simulink model "PFC_69C_03_06_V01_3Phase_3_2KW"  (R2022b)
settings: Solver=FixedStepAuto  StartTime=0.0  StopTime=Inf  RelTol=1e-3  EnableMultiTasking=on
model workspace (MAT data in the model file):
  ADC_Gain = 1241.21212121
  DAC_Gain = 0.000805860805861
  Inductor_Current_Divider_Gain_Phase_A = 33.4
  Inductor_Current_Divider_Gain_Phase_B = 33.4
  Vbulk_Divider_Gain = 276.854928018
  Vin_Divider_Gain = 556.17352614
undefined symbols (not defined in the file or in its folder): GPTRIP1SEL, GPTRIP2SEL, SCI_A_Transmit, SCI_A_Transmit_Current_Suffix, SCI_A_Transmit_one_shot_Suffix, SCI_A_Transmit_Polarity_Suffix, SCI_A_Transmit_relay_Suffix, SCI_A_Transmit_Vbulk_Suffix, SCI_A_Transmit_Vin_rms_Suffix, SCI_A_Transmit_Vin_Suffix, SCI_A_Transmit_Vmid_Suffix, SCI_A_Transmit_Vp_Suffix, SCI_A_Transmit_Vpfc_Suffix, TZ1, TZ2
libraries: c280xlib x38, c2802xlib x34, simulink x17, c2000lib x1
(part 2 of 8)

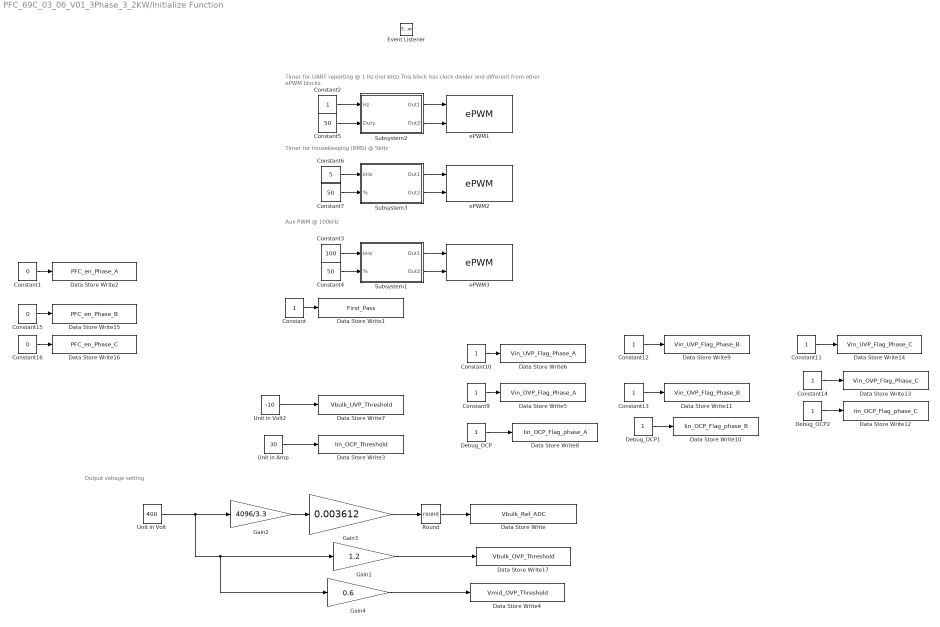
== system PFC_69C_03_06_V01_3Phase_3_2KW/Initialize Function ==
  note: Aux PWM @ 100kHz
  note: Timer for UART reporting @ 1 Hz (not kHz)
      | This block has clock divider and different from other ePWM blocks.
  note: Timer for housekeeping (RMS) @ 5kHz
  note: Output voltage setting
  Constant{,2,9..14} (8 alike) : Constant
  Constant1 : Constant  Value=0
  Constant15 : Constant  Value=0
  Constant16 : Constant  Value=0
  Constant3 : Constant  Value=100
  Constant4 : Constant  Value=50
  Constant5 : Constant  Value=50
  Constant6 : Constant  Value=5
  Constant7 : Constant  Value=50
  Data Store Write : DataStoreWrite  DataStoreName=Vbulk_Ref_ADC  IndexOptions=Index vector (dialog)  Indices=1  OutputSizes=1
  Data Store Write1 : DataStoreWrite  DataStoreName=First_Pass  IndexOptions=Index vector (dialog)  Indices=1  OutputSizes=1
  Data Store Write10 : DataStoreWrite  DataStoreName=Iin_OCP_Flag_phase_B  IndexOptions=Index vector (dialog)  Indices=1  OutputSizes=1
  Data Store Write11 : DataStoreWrite  DataStoreName=Vin_OVP_Flag_Phase_B  IndexOptions=Index vector (dialog)  Indices=1  OutputSizes=1
  Data Store Write12 : DataStoreWrite  DataStoreName=Iin_OCP_Flag_phase_C  IndexOptions=Index vector (dialog)  Indices=1  OutputSizes=1
  Data Store Write13 : DataStoreWrite  DataStoreName=Vin_OVP_Flag_Phase_C  IndexOptions=Index vector (dialog)  Indices=1  OutputSizes=1
  Data Store Write14 : DataStoreWrite  DataStoreName=Vin_UVP_Flag_Phase_C  IndexOptions=Index vector (dialog)  Indices=1  OutputSizes=1
  Data Store Write15 : DataStoreWrite  DataStoreName=PFC_en_Phase_B  IndexOptions=Index vector (dialog)  Indices=1  OutputSizes=1
  Data Store Write16 : DataStoreWrite  DataStoreName=PFC_en_Phase_C  IndexOptions=Index vector (dialog)  Indices=1  OutputSizes=1
  Data Store Write17 : DataStoreWrite  DataStoreName=Vbulk_OVP_Threshold  IndexOptions=Index vector (dialog)  Indices=1  OutputSizes=1
  Data Store Write2 : DataStoreWrite  DataStoreName=PFC_en_Phase_A  IndexOptions=Index vector (dialog)  Indices=1  OutputSizes=1
  Data Store Write3 : DataStoreWrite  DataStoreName=Iin_OCP_Threshold  IndexOptions=Index vector (dialog)  Indices=1  OutputSizes=1
  Data Store Write4 : DataStoreWrite  DataStoreName=Vmid_OVP_Threshold  IndexOptions=Index vector (dialog)  Indices=1  OutputSizes=1
  Data Store Write5 : DataStoreWrite  DataStoreName=Vin_OVP_Flag_Phase_A  IndexOptions=Index vector (dialog)  Indices=1  OutputSizes=1
  Data Store Write6 : DataStoreWrite  DataStoreName=Vin_UVP_Flag_Phase_A  IndexOptions=Index vector (dialog)  Indices=1  OutputSizes=1
  Data Store Write7 : DataStoreWrite  DataStoreName=Vbulk_UVP_Threshold  IndexOptions=Index vector (dialog)  Indices=1  OutputSizes=1
  Data Store Write8 : DataStoreWrite  DataStoreName=Iin_OCP_Flag_phase_A  IndexOptions=Index vector (dialog)  Indices=1  OutputSizes=1
  Data Store Write9 : DataStoreWrite  DataStoreName=Vin_UVP_Flag_Phase_B  IndexOptions=Index vector (dialog)  Indices=1  OutputSizes=1
  Debug_OCP : Constant
  Debug_OCP1 : Constant
  Debug_OCP2 : Constant
  Event Listener : EventListener  DisableCoverage=on  EventName=reset
  Gain1 : Gain  Gain=1.2
  Gain2 : Gain  Gain=4096/3.3
  Gain3 : Gain  Gain=0.003612  OutDataTypeStr=double
  Gain4 : Gain  Gain=0.6
  Round : Rounding  Operator=round
  Subsystem1 : Subsystem
  Subsystem2 : Subsystem
  Subsystem3 : Subsystem
  Unit in Amp : Constant  Value=30
  Unit in Volt : Constant  Value=400
  Unit in Volt2 : Constant  Value=-10
  ePWM1 : c2802xlib/ePWM  PwmType=C2000  useModule=ePWM7  ePWMxLINKTBPRD=Not Linked  periodUnits=Clock cycles  timerSource=Input port  timerPeriod_clk=50224  timerPeriod_sec=0.0001  tbshadow=Counter equals to zero  countingMode=Up  phaseActiveEnable=Disable  phaseDirection=Count down after sync  phaseActive=0  synchronizationEnable=off  dcaevt1Sync=off  dcbevt1Sync=off  synchronizationOption=Disable  dcbevt1SyncOut=off  dcaevt1SyncOut=off  cmpdSyncOut=off  cmpcSyncOut=off  cmpbSyncOut=off  zeroSyncOut=off  swfSyncOut=off  perSynchronizationOption=Counter equals to period (CTR=PRD)  clockPrescale=128  HSclockPrescale=14  enswap=off  ePWMxAStatus=on  ePWMxAactionLogic1=Clear  ePWMxAactionLogic2=Do nothing  ePWMxAactionLogic3=Set  ePWMxAactionLogic4=Set  ePWMxAactionLogic5=Do nothing  ePWMxAactionLogic6=Do nothing  ePWMxACSFenable=off  ePWMxACSFvalue=Forcing disable  ePWMxASFreload=Zero  ePWMxBStatus=off  ePWMxBactionLogic1=Set  ePWMxBactionLogic2=Do nothing  ePWMxBactionLogic3=Clear  ePWMxBactionLogic4=Do nothing  ePWMxBactionLogic5=Do nothing  ePWMxBactionLogic6=Set  ePWMxBCSFenable=off  ePWMxBCSFvalue=Forcing disable  ePWMxBSFreload=Zero  ePWNxBOutWay=off  ePWMxLINKCMPA=Not Linked  CMPAUnits=Clock cycles  CMPASource=Input port  CMPAValue_per=50  CMPAValue_clk=32000  enCMPAshadow=Counter equals to zero (CTR=Zero)  ePWMxLINKCMPB=Not Linked  CMPBUnits=Clock cycles  CMPBSource=Specify via dialog  CMPBValue_per=50  CMPBValue_clk=32000  enCMPBshadow=Counter equals to zero (CTR=Zero)  ePWMxLINKCMPC=Not Linked  CMPCUnits=Clock cycles  CMPCSource=Specify via dialog  CMPCValue_per=50  CMPCValue_clk=32000  enCMPCshadow=Counter equals to zero (CTR=Zero)  ePWMxLINKCMPD=Not Linked  CMPDUnits=Clock cycles  CMPDSource=Specify via dialog  CMPDValue_per=50  CMPDValue_clk=32000  enCMPDshadow=Counter equals to zero (CTR=Zero)  enableDBePWMxA=off  enableDBePWMxB=off  enhalfcycle=off  DBpolarity=Active high (AH)  DBedgeDelay=Positive  DBSource_ePWMxA=ePWMxA  DBSource_ePWMxB=ePWMxA  DBPeriodUnits=Clock cycles  DBperiodSource=Specify via dialog  REDperiod=0  FEDperiod=0  REDperiod_sec=0  FEDperiod_sec=0  LoadModeDBRED=Immediate without using shadow  LoadModeDBFED=Immediate without using shadow  adcstartModuleA=off  adcrequestEventA=First event  adcstartEventA=Counter equals to zero (CTR=Zero)  adcstartEventA_type2=Digital Compare Module A Event 1 start of conversion (DCAEVT1.soc)  adcstartModuleB=off  adcrequestEventB=First event  adcstartEventB=Counter equals to zero (CTR=Zero)  adcstartEventB_type2=Counter equals to zero (CTR=Zero)  intEn=on  intPrd=First event  intSel=Counter equals to zero (CTR=Zero)  intSel_type2=Counter equals to zero (CTR=Zero)  hrpe=off  enHRPWM=off  HRPWM_LoadMode=Counter equals to period (CTR=PRD)  HRPWM_CTLMode=Duty or Period control mode  HRPWM_EDGMode=Both edge  hrpeb=off  enHRPWMB=off  HRPWM_LoadModeB=Counter equals to zero (CTR=ZERO)  HRPWM_CTLModeB=Duty or Period control mode  HRPWM_EDGModeB=Both edge  enHRDBRED=off  enHRDBFED=off  enSFO=on  enautoconv=on  chopperEnable=off  chopperFrequency=1  chopperFirstwidth=1  chopperDuty=12.5%  tripZonesource=Specify via dialog  tzselOSHT1=off  tzselOSHT2=off  tzselOSHT3=off  tzselOSHDCAEV1=off  tzselOSHDCBEV1=off  tzselCBC1=off  tzselCBC2=off  tzselCBC3=off  tzselCBCDCAEV2=off  tzselCBCDCBEV2=off  tzselOSHT4=off  tzselOSHT5=off  tzselOSHT6=off  tzselCBC4=off  tzselCBC5=off  tzselCBC6=off  enTzOstIntr=off  enTzCbcIntr=off  enTzDCAEVT1Intr=off  enTzDCAEVT2Intr=off  enTzDCBEVT1Intr=off  enTzDCBEVT2Intr=off  ePWMxAforced=No action  ePWMxBforced=No action  DCAEVT1forced=No action  DCBEVT1forced=No action  DCAEVT2forced=No action  DCBEVT2forced=No action  dcah=Trip Zone 1 input (TZ1)  dcal=Trip Zone 1 input (TZ1)  dcbh=Trip Zone 1 input (TZ1)  dcbl=Trip Zone 1 input (TZ1)  dcah_type2=GPTRIP1SEL/(TZ1)  dcal_type2=GPTRIP2SEL/(TZ2)  dcbh_type2=GPTRIP1SEL/(TZ1)  dcbl_type2=GPTRIP2SEL/(TZ2)  gendcaevt1=Event disabled  gendcaevt2=Event disabled  gendcbevt1=Event disabled  gendcbevt2=Event disabled  dcaevt1src=DCAEVT1 with sync  dcaevt2src=DCAEVT2 with sync  dcbevt1src=DCBEVT1 with sync  dcbevt2src=DCBEVT2 with sync  pulsesel=Counter equals to zero (CTR=Zero)  blankinv=off  blankoffset=0  blankwidth=0  evsrcsel=Filtered version of DCAEVT1 (DCAEVT1FILT)  encape=off
      settings: LibrarySourceBlock=c2806xlib/ePWM
  ePWM2 : c2802xlib/ePWM  PwmType=C2000  useModule=ePWM4  ePWMxLINKTBPRD=Not Linked  periodUnits=Clock cycles  timerSource=Input port  timerPeriod_clk=64000  timerPeriod_sec=0.0001  tbshadow=Counter equals to zero  countingMode=Up  phaseActiveEnable=Disable  phaseDirection=Count down after sync  phaseActive=0  synchronizationEnable=off  dcaevt1Sync=off  dcbevt1Sync=off  synchronizationOption=Disable  dcbevt1SyncOut=off  dcaevt1SyncOut=off  cmpdSyncOut=off  cmpcSyncOut=off  cmpbSyncOut=off  zeroSyncOut=off  swfSyncOut=off  perSynchronizationOption=Counter equals to period (CTR=PRD)  clockPrescale=1  HSclockPrescale=1  enswap=off  ePWMxAStatus=on  ePWMxAactionLogic1=Clear  ePWMxAactionLogic2=Do nothing  ePWMxAactionLogic3=Set  ePWMxAactionLogic4=Set  ePWMxAactionLogic5=Do nothing  ePWMxAactionLogic6=Do nothing  ePWMxACSFenable=off  ePWMxACSFvalue=Forcing disable  ePWMxASFreload=Zero  ePWMxBStatus=off  ePWMxBactionLogic1=Set  ePWMxBactionLogic2=Do nothing  ePWMxBactionLogic3=Clear  ePWMxBactionLogic4=Do nothing  ePWMxBactionLogic5=Do nothing  ePWMxBactionLogic6=Set  ePWMxBCSFenable=off  ePWMxBCSFvalue=Forcing disable  ePWMxBSFreload=Zero  ePWNxBOutWay=off  ePWMxLINKCMPA=Not Linked  CMPAUnits=Clock cycles  CMPASource=Input port  CMPAValue_per=50  CMPAValue_clk=32000  enCMPAshadow=Counter equals to zero (CTR=Zero)  ePWMxLINKCMPB=Not Linked  CMPBUnits=Clock cycles  CMPBSource=Specify via dialog  CMPBValue_per=50  CMPBValue_clk=32000  enCMPBshadow=Counter equals to zero (CTR=Zero)  ePWMxLINKCMPC=Not Linked  CMPCUnits=Clock cycles  CMPCSource=Specify via dialog  CMPCValue_per=50  CMPCValue_clk=32000  enCMPCshadow=Counter equals to zero (CTR=Zero)  ePWMxLINKCMPD=Not Linked  CMPDUnits=Clock cycles  CMPDSource=Specify via dialog  CMPDValue_per=50  CMPDValue_clk=32000  enCMPDshadow=Counter equals to zero (CTR=Zero)  enableDBePWMxA=off  enableDBePWMxB=off  enhalfcycle=off  DBpolarity=Active high (AH)  DBedgeDelay=Positive  DBSource_ePWMxA=ePWMxA  DBSource_ePWMxB=ePWMxA  DBPeriodUnits=Clock cycles  DBperiodSource=Specify via dialog  REDperiod=0  FEDperiod=0  REDperiod_sec=0  FEDperiod_sec=0  LoadModeDBRED=Immediate without using shadow  LoadModeDBFED=Immediate without using shadow  adcstartModuleA=off  adcrequestEventA=First event  adcstartEventA=Counter equals to zero (CTR=Zero)  adcstartEventA_type2=Digital Compare Module A Event 1 start of conversion (DCAEVT1.soc)  adcstartModuleB=off  adcrequestEventB=First event  adcstartEventB=Counter equals to zero (CTR=Zero)  adcstartEventB_type2=Counter equals to zero (CTR=Zero)  intEn=on  intPrd=First event  intSel=Counter equals to zero (CTR=Zero)  intSel_type2=Counter equals to zero (CTR=Zero)  hrpe=off  enHRPWM=off  HRPWM_LoadMode=Counter equals to period (CTR=PRD)  HRPWM_CTLMode=Duty or Period control mode  HRPWM_EDGMode=Both edge  hrpeb=off  enHRPWMB=off  HRPWM_LoadModeB=Counter equals to zero (CTR=ZERO)  HRPWM_CTLModeB=Duty or Period control mode  HRPWM_EDGModeB=Both edge  enHRDBRED=off  enHRDBFED=off  enSFO=on  enautoconv=on  chopperEnable=off  chopperFrequency=1  chopperFirstwidth=1  chopperDuty=12.5%  tripZonesource=Specify via dialog  tzselOSHT1=off  tzselOSHT2=off  tzselOSHT3=off  tzselOSHDCAEV1=off  tzselOSHDCBEV1=off  tzselCBC1=off  tzselCBC2=off  tzselCBC3=off  tzselCBCDCAEV2=off  tzselCBCDCBEV2=off  tzselOSHT4=off  tzselOSHT5=off  tzselOSHT6=off  tzselCBC4=off  tzselCBC5=off  tzselCBC6=off  enTzOstIntr=off  enTzCbcIntr=off  enTzDCAEVT1Intr=off  enTzDCAEVT2Intr=off  enTzDCBEVT1Intr=off  enTzDCBEVT2Intr=off  ePWMxAforced=No action  ePWMxBforced=No action  DCAEVT1forced=No action  DCBEVT1forced=No action  DCAEVT2forced=No action  DCBEVT2forced=No action  dcah=Trip Zone 1 input (TZ1)  dcal=Trip Zone 1 input (TZ1)  dcbh=Trip Zone 1 input (TZ1)  dcbl=Trip Zone 1 input (TZ1)  dcah_type2=GPTRIP1SEL/(TZ1)  dcal_type2=GPTRIP2SEL/(TZ2)  dcbh_type2=GPTRIP1SEL/(TZ1)  dcbl_type2=GPTRIP2SEL/(TZ2)  gendcaevt1=Event disabled  gendcaevt2=Event disabled  gendcbevt1=Event disabled  gendcbevt2=Event disabled  dcaevt1src=DCAEVT1 with sync  dcaevt2src=DCAEVT2 with sync  dcbevt1src=DCBEVT1 with sync  dcbevt2src=DCBEVT2 with sync  pulsesel=Counter equals to zero (CTR=Zero)  blankinv=off  blankoffset=0  blankwidth=0  evsrcsel=Filtered version of DCAEVT1 (DCAEVT1FILT)  encape=off
      settings: LibrarySourceBlock=c2806xlib/ePWM
  ePWM3 : c2802xlib/ePWM  PwmType=C2000  useModule=ePWM8  ePWMxLINKTBPRD=Not Linked  periodUnits=Clock cycles  timerSource=Input port  timerPeriod_clk=64000  timerPeriod_sec=0.0001  tbshadow=Counter equals to zero  countingMode=Up  phaseActiveEnable=Disable  phaseDirection=Count down after sync  phaseActive=0  synchronizationEnable=off  dcaevt1Sync=off  dcbevt1Sync=off  synchronizationOption=Disable  dcbevt1SyncOut=off  dcaevt1SyncOut=off  cmpdSyncOut=off  cmpcSyncOut=off  cmpbSyncOut=off  zeroSyncOut=off  swfSyncOut=off  perSynchronizationOption=Counter equals to period (CTR=PRD)  clockPrescale=1  HSclockPrescale=1  enswap=off  ePWMxAStatus=on  ePWMxAactionLogic1=Clear  ePWMxAactionLogic2=Do nothing  ePWMxAactionLogic3=Set  ePWMxAactionLogic4=Set  ePWMxAactionLogic5=Do nothing  ePWMxAactionLogic6=Do nothing  ePWMxACSFenable=off  ePWMxACSFvalue=Forcing disable  ePWMxASFreload=Zero  ePWMxBStatus=on  ePWMxBactionLogic1=Set  ePWMxBactionLogic2=Do nothing  ePWMxBactionLogic3=Clear  ePWMxBactionLogic4=Do nothing  ePWMxBactionLogic5=Do nothing  ePWMxBactionLogic6=Set  ePWMxBCSFenable=off  ePWMxBCSFvalue=Forcing disable  ePWMxBSFreload=Zero  ePWNxBOutWay=off  ePWMxLINKCMPA=Not Linked  CMPAUnits=Clock cycles  CMPASource=Input port  CMPAValue_per=50  CMPAValue_clk=32000  enCMPAshadow=Counter equals to zero (CTR=Zero)  ePWMxLINKCMPB=Not Linked  CMPBUnits=Clock cycles  CMPBSource=Specify via dialog  CMPBValue_per=50  CMPBValue_clk=32000  enCMPBshadow=Counter equals to zero (CTR=Zero)  ePWMxLINKCMPC=Not Linked  CMPCUnits=Clock cycles  CMPCSource=Specify via dialog  CMPCValue_per=50  CMPCValue_clk=32000  enCMPCshadow=Counter equals to zero (CTR=Zero)  ePWMxLINKCMPD=Not Linked  CMPDUnits=Clock cycles  CMPDSource=Specify via dialog  CMPDValue_per=50  CMPDValue_clk=32000  enCMPDshadow=Counter equals to zero (CTR=Zero)  enableDBePWMxA=off  enableDBePWMxB=off  enhalfcycle=off  DBpolarity=Active high (AH)  DBedgeDelay=Positive  DBSource_ePWMxA=ePWMxA  DBSource_ePWMxB=ePWMxA  DBPeriodUnits=Clock cycles  DBperiodSource=Specify via dialog  REDperiod=0  FEDperiod=0  REDperiod_sec=0  FEDperiod_sec=0  LoadModeDBRED=Immediate without using shadow  LoadModeDBFED=Immediate without using shadow  adcstartModuleA=off  adcrequestEventA=First event  adcstartEventA=Counter equals to zero (CTR=Zero)  adcstartEventA_type2=Digital Compare Module A Event 1 start of conversion (DCAEVT1.soc)  adcstartModuleB=off  adcrequestEventB=First event  adcstartEventB=Counter equals to zero (CTR=Zero)  adcstartEventB_type2=Counter equals to zero (CTR=Zero)  intEn=off  intPrd=First event  intSel=Counter equals to zero (CTR=Zero)  intSel_type2=Counter equals to zero (CTR=Zero)  hrpe=off  enHRPWM=off  HRPWM_LoadMode=Counter equals to period (CTR=PRD)  HRPWM_CTLMode=Duty or Period control mode  HRPWM_EDGMode=Both edge  hrpeb=off  enHRPWMB=off  HRPWM_LoadModeB=Counter equals to zero (CTR=ZERO)  HRPWM_CTLModeB=Duty or Period control mode  HRPWM_EDGModeB=Both edge  enHRDBRED=off  enHRDBFED=off  enSFO=on  enautoconv=on  chopperEnable=off  chopperFrequency=1  chopperFirstwidth=1  chopperDuty=12.5%  tripZonesource=Specify via dialog  tzselOSHT1=off  tzselOSHT2=off  tzselOSHT3=off  tzselOSHDCAEV1=off  tzselOSHDCBEV1=off  tzselCBC1=off  tzselCBC2=off  tzselCBC3=off  tzselCBCDCAEV2=off  tzselCBCDCBEV2=off  tzselOSHT4=off  tzselOSHT5=off  tzselOSHT6=off  tzselCBC4=off  tzselCBC5=off  tzselCBC6=off  enTzOstIntr=off  enTzCbcIntr=off  enTzDCAEVT1Intr=off  enTzDCAEVT2Intr=off  enTzDCBEVT1Intr=off  enTzDCBEVT2Intr=off  ePWMxAforced=No action  ePWMxBforced=No action  DCAEVT1forced=No action  DCBEVT1forced=No action  DCAEVT2forced=No action  DCBEVT2forced=No action  dcah=Trip Zone 1 input (TZ1)  dcal=Trip Zone 1 input (TZ1)  dcbh=Trip Zone 1 input (TZ1)  dcbl=Trip Zone 1 input (TZ1)  dcah_type2=GPTRIP1SEL/(TZ1)  dcal_type2=GPTRIP2SEL/(TZ2)  dcbh_type2=GPTRIP1SEL/(TZ1)  dcbl_type2=GPTRIP2SEL/(TZ2)  gendcaevt1=Event disabled  gendcaevt2=Event disabled  gendcbevt1=Event disabled  gendcbevt2=Event disabled  dcaevt1src=DCAEVT1 with sync  dcaevt2src=DCAEVT2 with sync  dcbevt1src=DCBEVT1 with sync  dcbevt2src=DCBEVT2 with sync  pulsesel=Counter equals to zero (CTR=Zero)  blankinv=off  blankoffset=0  blankwidth=0  evsrcsel=Filtered version of DCAEVT1 (DCAEVT1FILT)  encape=off
      settings: LibrarySourceBlock=c2806xlib/ePWM
  wires:
  Constant6/1 -> Subsystem3/1(kHz)
  Constant7/1 -> Subsystem3/2(%)
  Constant4/1 -> Subsystem1/2(%)
  Subsystem1/1(Out1) -> ePWM3/1
  Constant2/1 -> Subsystem2/1(Hz)
  Subsystem3/2(Out2) -> ePWM2/2
  Subsystem3/1(Out1) -> ePWM2/1
  Constant3/1 -> Subsystem1/1(kHz)
  Constant5/1 -> Subsystem2/2(Duty)
  Subsystem2/1(Out1) -> ePWM1/1
  Subsystem1/2(Out2) -> ePWM3/2
  Subsystem2/2(Out2) -> ePWM1/2
  Constant/1 -> Data Store Write1/1
  Constant1/1 -> Data Store Write2/1
  Gain2/1 -> Gain3/1
  Constant9/1 -> Data Store Write5/1
  Constant10/1 -> Data Store Write6/1
  Unit in Volt2/1 -> Data Store Write7/1
  Unit in Amp/1 -> Data Store Write3/1
  Debug_OCP/1 -> Data Store Write8/1
  Gain3/1 -> Round/1
  Round/1 -> Data Store Write/1
  Constant12/1 -> Data Store Write9/1
  Debug_OCP1/1 -> Data Store Write10/1
  Constant13/1 -> Data Store Write11/1
  Debug_OCP2/1 -> Data Store Write12/1
  Constant14/1 -> Data Store Write13/1
  Constant11/1 -> Data Store Write14/1
  Constant15/1 -> Data Store Write15/1
  Constant16/1 -> Data Store Write16/1
  Gain1/1 -> Data Store Write17/1
  Unit in Volt/1 -> Gain4/1, Gain1/1, Gain2/1
  Gain4/1 -> Data Store Write4/1

== system PFC_69C_03_06_V01_3Phase_3_2KW/Initialize ePWM1 ==

== system PFC_69C_03_06_V01_3Phase_3_2KW/PWM Update @50KHz ==
  note: This block will update PWM after control calculations.==>
  function : TriggerPort  TriggerType=function-call  VariantControl=(inherit)
  Current loop PWM generation (Control) : Subsystem  TreatAsAtomicUnit=on
  Fixed Duty update_Phase_A : Subsystem  TreatAsAtomicUnit=on
  Fixed Duty update_Phase_B_Test : Subsystem  TreatAsAtomicUnit=on
  Fixed Duty update_Phase_C : Subsystem  TreatAsAtomicUnit=on
  Function-Call Generator : simulink/Ports & Subsystems/Function-Call Generator  sample_time=-1  numberOfIterations=1  DisallowWideOutput=off
  Function-Call Split : FunctionCallSplit  IconShape=distinctive  NumOutputPorts=5  OutputPortLayout=default
  Voltage loop PWM generation (Control) : Subsystem  Commented=on  TreatAsAtomicUnit=on
  wires:
  Function-Call Generator/1 -> Function-Call Split/1
  Function-Call Split/5 -> Fixed Duty update_Phase_C/Trigger
  Function-Call Split/4 -> Fixed Duty update_Phase_B_Test/Trigger
  Function-Call Split/3 -> Fixed Duty update_Phase_A/Trigger
  Function-Call Split/2 -> Current loop PWM generation (Control)/Trigger
  Function-Call Split/1 -> Voltage loop PWM generation (Control)/Trigger

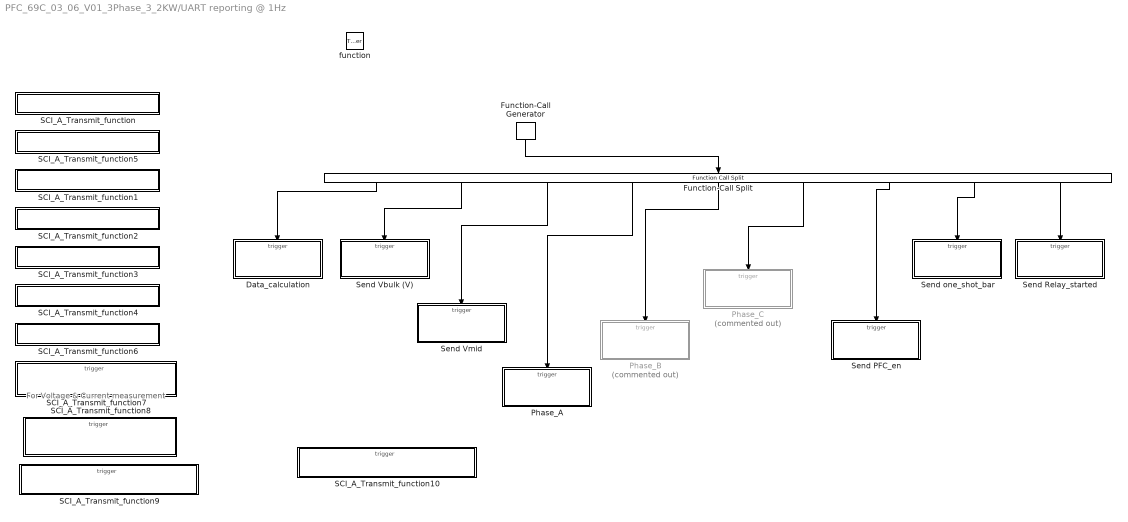
== system PFC_69C_03_06_V01_3Phase_3_2KW/UART reporting @ 1Hz ==
  note: For Voltage & Current measurement
  function : TriggerPort  TriggerType=function-call  VariantControl=(inherit)
  Data_calculation : Subsystem  TreatAsAtomicUnit=on
  Function-Call Generator : simulink/Ports & Subsystems/Function-Call Generator  sample_time=-1  numberOfIterations=1  DisallowWideOutput=off
  Function-Call Split : FunctionCallSplit  IconShape=distinctive  NumOutputPorts=9  OutputPortLayout=default
  Phase_A : Subsystem  TreatAsAtomicUnit=on
  Phase_B : Subsystem  Commented=on  TreatAsAtomicUnit=on
  Phase_C : Subsystem  Commented=on  TreatAsAtomicUnit=on
  SCI_A_Transmit_function : Subsystem  TreatAsAtomicUnit=on
  SCI_A_Transmit_function1 : Subsystem  TreatAsAtomicUnit=on
  SCI_A_Transmit_function10 : Subsystem  TreatAsAtomicUnit=on
  SCI_A_Transmit_function2 : Subsystem  TreatAsAtomicUnit=on
  SCI_A_Transmit_function3 : Subsystem  TreatAsAtomicUnit=on
  SCI_A_Transmit_function4 : Subsystem  TreatAsAtomicUnit=on
  SCI_A_Transmit_function5 : Subsystem  TreatAsAtomicUnit=on
  SCI_A_Transmit_function6 : Subsystem  TreatAsAtomicUnit=on
  SCI_A_Transmit_function7 : Subsystem  TreatAsAtomicUnit=on
  SCI_A_Transmit_function8 : Subsystem  TreatAsAtomicUnit=on
  SCI_A_Transmit_function9 : Subsystem  TreatAsAtomicUnit=on
  Send PFC_en : Subsystem  TreatAsAtomicUnit=on
  Send Relay_started : Subsystem  TreatAsAtomicUnit=on
  Send Vbulk (V) : Subsystem  TreatAsAtomicUnit=on
  Send Vmid : Subsystem  TreatAsAtomicUnit=on
  Send one_shot_bar : Subsystem  TreatAsAtomicUnit=on
  wires:
  Function-Call Split/2 -> Send Vbulk (V)/Trigger
  Function-Call Generator/1 -> Function-Call Split/1
  Function-Call Split/1 -> Data_calculation/Trigger
  Function-Call Split/3 -> Send Vmid/Trigger
  Function-Call Split/4 -> Phase_A/Trigger
  Function-Call Split/5 -> Phase_B/Trigger
  Function-Call Split/6 -> Phase_C/Trigger
  Function-Call Split/7 -> Send PFC_en/Trigger
  Function-Call Split/8 -> Send one_shot_bar/Trigger
  Function-Call Split/9 -> Send Relay_started/Trigger

== system PFC_69C_03_06_V01_3Phase_3_2KW/Calibration,RMS, Fault Protection @5kHz/Calibration ==
  function : TriggerPort  TriggerType=function-call  VariantControl=(inherit)
  Calibration_3phase : Subsystem  TreatAsAtomicUnit=on
  Calibration_Phase_A : Subsystem  TreatAsAtomicUnit=on
  Calibration_Phase_B : Subsystem  TreatAsAtomicUnit=on
  Calibration_Phase_C : Subsystem  TreatAsAtomicUnit=on
  Function-Call Generator : simulink/Ports & Subsystems/Function-Call Generator  sample_time=-1  numberOfIterations=1  DisallowWideOutput=off
  Function-Call Split : FunctionCallSplit  IconShape=distinctive  NumOutputPorts=4  OutputPortLayout=default
  wires:
  Function-Call Generator/1 -> Function-Call Split/1
  Function-Call Split/2 -> Calibration_Phase_B/Trigger
  Function-Call Split/1 -> Calibration_Phase_A/Trigger
  Function-Call Split/3 -> Calibration_Phase_C/Trigger
  Function-Call Split/4 -> Calibration_3phase/Trigger

== system PFC_69C_03_06_V01_3Phase_3_2KW/Calibration,RMS, Fault Protection @5kHz/Current_Control_REF_Adjusted_Phase_A ==
  function : TriggerPort  TriggerType=function-call  VariantControl=(inherit)
  Data Store Read20 : DataStoreRead  DataStoreName=Vbulk  IndexOptions=Index vector (dialog)  Indices=1  OutputSizes=1
  Data Store Read21 : DataStoreRead  DataStoreName=Vmid_Topside  IndexOptions=Index vector (dialog)  Indices=1  OutputSizes=1
  Data Store Read22 : DataStoreRead  DataStoreName=Control_Loop_Current_Phase_A  IndexOptions=Index vector (dialog)  Indices=1  OutputSizes=1
  Data Store Read23 : DataStoreRead  DataStoreName=Polarity_Phase_A  IndexOptions=Index vector (dialog)  Indices=1  OutputSizes=1
  Data Store Write6 : DataStoreWrite  DataStoreName=Ref_Loop_Current_Phase_A  IndexOptions=Index vector (dialog)  Indices=1  OutputSizes=1
  Mid Voltage Balancing_Ref_Current : Stateflow chart  TreatAsAtomicUnit=on
  wires:
  Data Store Read20/1 -> Mid Voltage Balancing_Ref_Current/1(VBulk)
  Data Store Read23/1 -> Mid Voltage Balancing_Ref_Current/2(Polarity_Phase_A)
  Data Store Read22/1 -> Mid Voltage Balancing_Ref_Current/4(Ref_Current_Phase_A)
  Mid Voltage Balancing_Ref_Current/1(output_y) -> Data Store Write6/1
  Data Store Read21/1 -> Mid Voltage Balancing_Ref_Current/3(Vmid)

== system PFC_69C_03_06_V01_3Phase_3_2KW/Calibration,RMS, Fault Protection @5kHz/Current_Control_REF_Adjusted_Phase_B ==
  function : TriggerPort  TriggerType=function-call  VariantControl=(inherit)
  Data Store Read20 : DataStoreRead  DataStoreName=Vbulk  IndexOptions=Index vector (dialog)  Indices=1  OutputSizes=1
  Data Store Read21 : DataStoreRead  DataStoreName=Vmid_Topside  IndexOptions=Index vector (dialog)  Indices=1  OutputSizes=1
  Data Store Read22 : DataStoreRead  DataStoreName=Control_Loop_Current_Phase_B  IndexOptions=Index vector (dialog)  Indices=1  OutputSizes=1
  Data Store Read23 : DataStoreRead  DataStoreName=Polarity_Phase_B  IndexOptions=Index vector (dialog)  Indices=1  OutputSizes=1
  Data Store Write6 : DataStoreWrite  DataStoreName=Ref_Loop_Current_Phase_B  IndexOptions=Index vector (dialog)  Indices=1  OutputSizes=1
  Mid Voltage Balancing_Ref_Current : Stateflow chart  TreatAsAtomicUnit=on
  wires:
  Data Store Read20/1 -> Mid Voltage Balancing_Ref_Current/1(VBulk)
  Data Store Read23/1 -> Mid Voltage Balancing_Ref_Current/2(Polarity_Phase_A)
  Data Store Read22/1 -> Mid Voltage Balancing_Ref_Current/4(Ref_Current_Phase_A)
  Mid Voltage Balancing_Ref_Current/1(output_y) -> Data Store Write6/1
  Data Store Read21/1 -> Mid Voltage Balancing_Ref_Current/3(Vmid)

== system PFC_69C_03_06_V01_3Phase_3_2KW/Calibration,RMS, Fault Protection @5kHz/Current_Control_REF_Adjusted_Phase_C ==
  function : TriggerPort  TriggerType=function-call  VariantControl=(inherit)
  Data Store Read20 : DataStoreRead  DataStoreName=Vbulk  IndexOptions=Index vector (dialog)  Indices=1  OutputSizes=1
  Data Store Read21 : DataStoreRead  DataStoreName=Vmid_Topside  IndexOptions=Index vector (dialog)  Indices=1  OutputSizes=1
  Data Store Read22 : DataStoreRead  DataStoreName=Control_Loop_Current_Phase_C  IndexOptions=Index vector (dialog)  Indices=1  OutputSizes=1
  Data Store Read23 : DataStoreRead  DataStoreName=Polarity_Phase_C  IndexOptions=Index vector (dialog)  Indices=1  OutputSizes=1
  Data Store Write6 : DataStoreWrite  DataStoreName=Ref_Loop_Current_Phase_C  IndexOptions=Index vector (dialog)  Indices=1  OutputSizes=1
  Mid Voltage Balancing_Ref_Current : Stateflow chart  TreatAsAtomicUnit=on
  wires:
  Data Store Read20/1 -> Mid Voltage Balancing_Ref_Current/1(VBulk)
  Data Store Read23/1 -> Mid Voltage Balancing_Ref_Current/2(Polarity_Phase_A)
  Data Store Read22/1 -> Mid Voltage Balancing_Ref_Current/4(Ref_Current_Phase_A)
  Mid Voltage Balancing_Ref_Current/1(output_y) -> Data Store Write6/1
  Data Store Read21/1 -> Mid Voltage Balancing_Ref_Current/3(Vmid)

== system PFC_69C_03_06_V01_3Phase_3_2KW/Calibration,RMS, Fault Protection @5kHz/Fault checking ==
  function : TriggerPort  TriggerType=function-call  VariantControl=(inherit)
  Data Store Read4 : DataStoreRead  DataStoreName=Calibration_Done  IndexOptions=Index vector (dialog)  Indices=1  OutputSizes=1
  If : If  IfExpression=u1 ==1  ShowElse=off
  If Action Subsystem : Subsystem  TreatAsAtomicUnit=on
  wires:
  If/1 -> If Action Subsystem/Action
  Data Store Read4/1 -> If/1

== system PFC_69C_03_06_V01_3Phase_3_2KW/Calibration,RMS, Fault Protection @5kHz/PFC_en and output//input ==
  function : TriggerPort  TriggerType=function-call  VariantControl=(inherit)
  Chart1 : Stateflow chart  TreatAsAtomicUnit=on
      settings: PortSchema="{\"entries\":[{\"content\":{\"sides\":[{\"content\":{\"connectorIds\":[]},\"type\":\"ConnectorPlacement.EquallySpacedRectSide\",\"uuid\":\"98054acb-dc05-45b7-9e49-d1f1309a60af\"},{\"content\":{\"connectorIds\":[\"Out1\",\"Out2\",\"Out3\",\"Out4\"],\"side\":\"RIGHT\"},\"type\":\"ConnectorPlacement.EquallySpacedRectSide\",\"uuid\":\"519c6a11-fba4-4420-9bc2-f24cec898983\"},{\"content\":{\"connectorIds\":[\"In1\"],\"side\":\"TOP\"},\"type\":\"ConnectorPlacement.EquallySpacedRectSide\",\"uuid\":\"37e92206-8070-4c6c-85b3-8eb12c5538cd\"},{\"content\":{\"connectorIds\":[],\"side\":\"BOTTOM\"},\"type\":\"ConnectorPlacement.EquallySpacedRectSide\",\"uuid\":\"a24e42b6-e88f-4c7d-a70a-f75d0d02a985\"}]},\"type\":\"ConnectorPlacement.EquallySpacedConnector\",\"uuid\":\"7d467722-ac20-43d4-98e5-7341f60d2894\"}],\"packageUris\":[\"http://schema.mathworks.com/mf0/Connector/R2020b\"],\"version\":\"1.0\"}"
  Data Store Read7 : DataStoreRead  DataStoreName=PFC_en  IndexOptions=Index vector (dialog)  Indices=1  OutputSizes=1
  Data Store Write : DataStoreWrite  DataStoreName=input_z1  IndexOptions=Index vector (dialog)  Indices=1  OutputSizes=1
  Data Store Write1 : DataStoreWrite  DataStoreName=input_z2  IndexOptions=Index vector (dialog)  Indices=1  OutputSizes=1
  Data Store Write2 : DataStoreWrite  DataStoreName=output_z1  IndexOptions=Index vector (dialog)  Indices=1  OutputSizes=1
  Data Store Write3 : DataStoreWrite  DataStoreName=output_z2  IndexOptions=Index vector (dialog)  Indices=1  OutputSizes=1
  wires:
  Data Store Read7/1 -> Chart1/1(PFC_en)
  Chart1/1(input_z1) -> Data Store Write/1
  Chart1/4(input_z2) -> Data Store Write1/1
  Chart1/2(output_z1) -> Data Store Write2/1
  Chart1/3(output_z2) -> Data Store Write3/1

== system PFC_69C_03_06_V01_3Phase_3_2KW/Calibration,RMS, Fault Protection @5kHz/Polarity & Near Zero check ==
  function : TriggerPort  TriggerType=function-call  VariantControl=(inherit)
  Function-Call Generator : simulink/Ports & Subsystems/Function-Call Generator  sample_time=-1  numberOfIterations=1  DisallowWideOutput=off
  Function-Call Split : FunctionCallSplit  IconShape=distinctive  NumOutputPorts=3  OutputPortLayout=default
  Polarity_Near_zero_Phase_A : Subsystem  TreatAsAtomicUnit=on
  Polarity_Near_zero_Phase_B : Subsystem  TreatAsAtomicUnit=on
  Polarity_Near_zero_Phase_C : Subsystem  TreatAsAtomicUnit=on
  wires:
  Function-Call Generator/1 -> Function-Call Split/1
  Function-Call Split/1 -> Polarity_Near_zero_Phase_A/Trigger
  Function-Call Split/2 -> Polarity_Near_zero_Phase_B/Trigger
  Function-Call Split/3 -> Polarity_Near_zero_Phase_C/Trigger

== system PFC_69C_03_06_V01_3Phase_3_2KW/Calibration,RMS, Fault Protection @5kHz/Relay control ==
  note: 0.2 x ms
  note: This block will be executed at every 1 mili second. (1kHz)
  function : TriggerPort  TriggerType=function-call  VariantControl=(inherit)
  ADC Gain : Subsystem
  Data Store Memory1 : DataStoreMemory  DataStoreName=RELAY_START_DELAY  WriteAfterWriteMsg=warning  ShowAdditionalParam=off
  Data Store Read1 : DataStoreRead  DataStoreName=RELAY_START_DELAY  IndexOptions=Index vector (dialog)  Indices=1  OutputSizes=1
  Data Store Read3 : DataStoreRead  DataStoreName=Vin_peak_ADC_Phase_A  IndexOptions=Index vector (dialog)  Indices=1  OutputSizes=1
  Data Store Read4 : DataStoreRead  DataStoreName=Relay_TurnON_Threshold  IndexOptions=Index vector (dialog)  Indices=1  OutputSizes=1
  Data Store Read5 : DataStoreRead  DataStoreName=PFC_en  IndexOptions=Index vector (dialog)  Indices=1  OutputSizes=1
  Data Store Write1 : DataStoreWrite  DataStoreName=RELAY_START_DELAY  IndexOptions=Index vector (dialog)  Indices=1  OutputSizes=1
  Data Store Write6 : DataStoreWrite  DataStoreName=Relay_started  IndexOptions=Index vector (dialog)  Indices=1  OutputSizes=1
  Relay_Control : Stateflow chart  TreatAsAtomicUnit=on
  Relay_GPIO1 : c280xlib/Digital Output  GPIO_Number=GPIO8~GPIO15  GPIO_Bit0=on  GPIO_BIT0_Toggle=off  GPIO_Bit1=off  GPIO_BIT1_Toggle=off  GPIO_Bit2=off  GPIO_BIT2_Toggle=off  GPIO_Bit3=off  GPIO_BIT3_Toggle=off  GPIO_Bit4=off  GPIO_BIT4_Toggle=off  GPIO_Bit5=off  GPIO_BIT5_Toggle=off  GPIO_Bit6=off  GPIO_BIT6_Toggle=off  GPIO_Bit7=off  GPIO_BIT7_Toggle=off
  Subsystem : Subsystem  Commented=on
  ms : Constant  Value=150
  wires:
  ADC Gain/1(Out1) -> Relay_Control/2(Relay_TurnON_Threshold_ADC)
  Data Store Read5/1 -> Relay_Control/4(PFC_en)
  ms/1 -> Data Store Write1/1
  Relay_Control/2(PWM_Turned_on) -> Data Store Write6/1
  Data Store Read4/1 -> ADC Gain/1(In1)
  Relay_Control/1(Relay_Started) -> Relay_GPIO1/1
  Data Store Read1/1 -> Relay_Control/3(RELAY_START_DELAY)
  Data Store Read3/1 -> Relay_Control/1(Vin_peak_ADC)

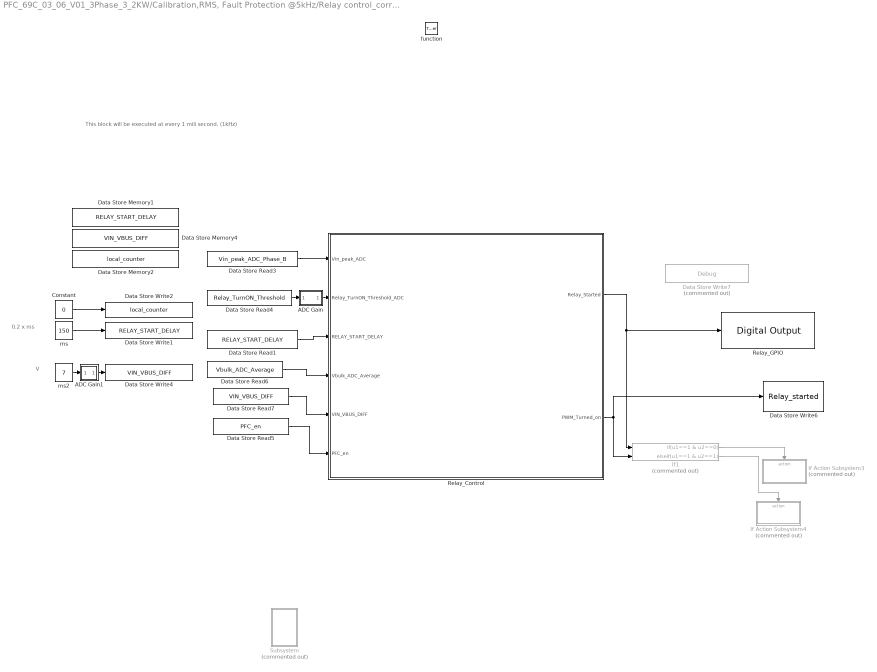
== system PFC_69C_03_06_V01_3Phase_3_2KW/Calibration,RMS, Fault Protection @5kHz/Relay control_corrected ==
  note: This block will be executed at every 1 mili second. (1kHz)
  note: 0.2 x ms
  note: V
  function : TriggerPort  TriggerType=function-call  VariantControl=(inherit)
  ADC Gain : Subsystem
  ADC Gain1 : Subsystem
  Constant : Constant  Value=0
  Data Store Memory1 : DataStoreMemory  DataStoreName=RELAY_START_DELAY  WriteAfterWriteMsg=warning  ShowAdditionalParam=off
  Data Store Memory2 : DataStoreMemory  DataStoreName=local_counter  WriteAfterWriteMsg=warning  ShowAdditionalParam=off
  Data Store Memory4 : DataStoreMemory  DataStoreName=VIN_VBUS_DIFF  WriteAfterWriteMsg=warning  ShowAdditionalParam=off
  Data Store Read1 : DataStoreRead  DataStoreName=RELAY_START_DELAY  IndexOptions=Index vector (dialog)  Indices=1  OutputSizes=1
  Data Store Read3 : DataStoreRead  DataStoreName=Vin_peak_ADC_Phase_B  IndexOptions=Index vector (dialog)  Indices=1  OutputSizes=1
  Data Store Read4 : DataStoreRead  DataStoreName=Relay_TurnON_Threshold  IndexOptions=Index vector (dialog)  Indices=1  OutputSizes=1
  Data Store Read5 : DataStoreRead  DataStoreName=PFC_en  IndexOptions=Index vector (dialog)  Indices=1  OutputSizes=1
  Data Store Read6 : DataStoreRead  DataStoreName=Vbulk_ADC_Average  IndexOptions=Index vector (dialog)  Indices=1  OutputSizes=1
  Data Store Read7 : DataStoreRead  DataStoreName=VIN_VBUS_DIFF  IndexOptions=Index vector (dialog)  Indices=1  OutputSizes=1
  Data Store Write1 : DataStoreWrite  DataStoreName=RELAY_START_DELAY  IndexOptions=Index vector (dialog)  Indices=1  OutputSizes=1
  Data Store Write2 : DataStoreWrite  DataStoreName=local_counter  IndexOptions=Index vector (dialog)  Indices=1  OutputSizes=1
  Data Store Write4 : DataStoreWrite  DataStoreName=VIN_VBUS_DIFF  IndexOptions=Index vector (dialog)  Indices=1  OutputSizes=1
  Data Store Write6 : DataStoreWrite  DataStoreName=Relay_started  IndexOptions=Index vector (dialog)  Indices=1  OutputSizes=1
  Data Store Write7 : DataStoreWrite  Commented=on  DataStoreName=Debug  IndexOptions=Index vector (dialog)  Indices=1  OutputSizes=1
  If Action Subsystem3 : Subsystem  Commented=on  TreatAsAtomicUnit=on
  If Action Subsystem4 : Subsystem  Commented=on  TreatAsAtomicUnit=on
  If1 : If  Commented=on  NumInputs=2  IfExpression=u1==1 & u2==0  ElseIfExpressions=u1==1 & u2==1  ShowElse=off
  Relay_Control : Stateflow chart  TreatAsAtomicUnit=on
  Relay_GPIO : c280xlib/Digital Output  GPIO_Number=GPIO8~GPIO15  GPIO_Bit0=on  GPIO_BIT0_Toggle=off  GPIO_Bit1=off  GPIO_BIT1_Toggle=off  GPIO_Bit2=off  GPIO_BIT2_Toggle=off  GPIO_Bit3=off  GPIO_BIT3_Toggle=off  GPIO_Bit4=off  GPIO_BIT4_Toggle=off  GPIO_Bit5=off  GPIO_BIT5_Toggle=off  GPIO_Bit6=off  GPIO_BIT6_Toggle=off  GPIO_Bit7=off  GPIO_BIT7_Toggle=off
  Subsystem : Subsystem  Commented=on
  ms : Constant  Value=150
  ms2 : Constant  Value=7
  wires:
  Relay_Control/2(PWM_Turned_on) -> If1/2, Data Store Write6/1
  Data Store Read6/1 -> Relay_Control/4(Vbulk_ADC_Average)
  Data Store Read7/1 -> Relay_Control/5(VIN_VBUS_DIFF)
  Data Store Read1/1 -> Relay_Control/3(RELAY_START_DELAY)
  ms/1 -> Data Store Write1/1
  If1/1 -> If Action Subsystem3/Action
  Data Store Read3/1 -> Relay_Control/1(Vin_peak_ADC)
  ADC Gain1/1(Out1) -> Data Store Write4/1
  ADC Gain/1(Out1) -> Relay_Control/2(Relay_TurnON_Threshold_ADC)
  Relay_Control/1(Relay_Started) -> If1/1, Relay_GPIO/1
  ms2/1 -> ADC Gain1/1(In1)
  Data Store Read4/1 -> ADC Gain/1(In1)
  Data Store Read5/1 -> Relay_Control/6(PFC_en)
  Constant/1 -> Data Store Write2/1
  If1/2 -> If Action Subsystem4/Action

== system PFC_69C_03_06_V01_3Phase_3_2KW/Calibration,RMS, Fault Protection @5kHz/Soft Start ==
  note: This will be used for control computation.
  function : TriggerPort  TriggerType=function-call  VariantControl=(inherit)
  Chart : Stateflow chart  TreatAsAtomicUnit=on
      settings: PortSchema="{\"entries\":[{\"content\":{\"sides\":[{\"content\":{\"connectorIds\":[\"In2\",\"In3\",\"In4\",\"In5\",\"In6\"]},\"type\":\"ConnectorPlacement.EquallySpacedRectSide\",\"uuid\":\"22b210d6-ceb6-4123-9311-ecfc1554a514\"},{\"content\":{\"connectorIds\":[\"Out2\",\"Out3\",\"Out4\"],\"side\":\"RIGHT\"},\"type\":\"ConnectorPlacement.EquallySpacedRectSide\",\"uuid\":\"bd71c4d7-1c84-49a9-97ae-3dc5e1ac2530\"},{\"content\":{\"connectorIds\":[\"In1\",\"Out1\"],\"side\":\"TOP\"},\"type\":\"ConnectorPlacement.EquallySpacedRectSide\",\"uuid\":\"720c9beb-f716-4abe-bf9b-a08f9ee3742e\"}]},\"type\":\"ConnectorPlacement.EquallySpacedConnector\",\"uuid\":\"ea96fba9-9c4e-4b61-9de0-918baa6c198f\"}],\"packageUris\":[\"http://schema.mathworks.com/mf0/Connector/R2020b\"],\"version\":\"1.0\"}"
  Data Store Read : DataStoreRead  DataStoreName=Relay_started  IndexOptions=Index vector (dialog)  Indices=1  OutputSizes=1
  Data Store Read1 : DataStoreRead  DataStoreName=Vbulk_ADC  IndexOptions=Index vector (dialog)  Indices=1  OutputSizes=1
  Data Store Read2 : DataStoreRead  DataStoreName=First_Pass  IndexOptions=Index vector (dialog)  Indices=1  OutputSizes=1
  Data Store Read3 : DataStoreRead  DataStoreName=Soft_Start  IndexOptions=Index vector (dialog)  Indices=1  OutputSizes=1
  Data Store Read4 : DataStoreRead  DataStoreName=Vbulk_Ref_ADC  IndexOptions=Index vector (dialog)  Indices=1  OutputSizes=1
  Data Store Read5 : DataStoreRead  DataStoreName=PFC_en  IndexOptions=Index vector (dialog)  Indices=1  OutputSizes=1
  Data Store Write : DataStoreWrite  DataStoreName=First_Pass  IndexOptions=Index vector (dialog)  Indices=1  OutputSizes=1
  Data Store Write2 : DataStoreWrite  DataStoreName=Vbulk_Ref_ADC_adjusted  IndexOptions=Index vector (dialog)  Indices=1  OutputSizes=1
  Data Store Write3 : DataStoreWrite  DataStoreName=Soft_Start  IndexOptions=Index vector (dialog)  Indices=1  OutputSizes=1
  wires:
  Data Store Read1/1 -> Chart/3(Vbulk_ADC)
  Data Store Read2/1 -> Chart/4("First_Pass ")
  Chart/2(First_Pass) -> Data Store Write/1
  Data Store Read3/1 -> Chart/5("Soft_Start ")
  Data Store Read4/1 -> Chart/6(Vbulk_Ref_ADC)
  Chart/4(Vbulk_Ref_ADC_adjusted) -> Data Store Write2/1
  Chart/3(Soft_Start) -> Data Store Write3/1
  Data Store Read5/1 -> Chart/2(PFC_en)
  Data Store Read/1 -> Chart/1(Relay_started)

== system PFC_69C_03_06_V01_3Phase_3_2KW/Calibration,RMS, Fault Protection @5kHz/Voltage RMS//Averag Calculation ==
  function : TriggerPort  TriggerType=function-call  VariantControl=(inherit)
  Function-Call Generator : simulink/Ports & Subsystems/Function-Call Generator  sample_time=-1  numberOfIterations=1  DisallowWideOutput=off
  Function-Call Split : FunctionCallSplit  IconShape=distinctive  NumOutputPorts=5  OutputPortLayout=default
  Phase_A : Subsystem  TreatAsAtomicUnit=on
  Phase_B : Subsystem  TreatAsAtomicUnit=on
  Phase_C : Subsystem  TreatAsAtomicUnit=on
  Vbulk_ADC Averaging : Subsystem  TreatAsAtomicUnit=on
  Vmid_ADC Averaging : Subsystem  TreatAsAtomicUnit=on
  wires:
  Function-Call Generator/1 -> Function-Call Split/1
  Function-Call Split/1 -> Vbulk_ADC Averaging/Trigger
  Function-Call Split/5 -> Phase_C/Trigger
  Function-Call Split/4 -> Phase_B/Trigger
  Function-Call Split/3 -> Phase_A/Trigger
  Function-Call Split/2 -> Vmid_ADC Averaging/Trigger

== system PFC_69C_03_06_V01_3Phase_3_2KW/Calibration,RMS, Fault Protection @5kHz/Voltage loop PWM generation (Control) ==
  function : TriggerPort  TriggerType=function-call  VariantControl=(inherit)
  Data Store Read1 : DataStoreRead  DataStoreName=Relay_started  IndexOptions=Index vector (dialog)  Indices=1  OutputSizes=1
  Data Store Read7 : DataStoreRead  DataStoreName=PFC_en  IndexOptions=Index vector (dialog)  Indices=1  OutputSizes=1
  If : If  NumInputs=2  IfExpression=(u1==1) & (u2==1)  ShowElse=off
  If Action Subsystem : Subsystem  TreatAsAtomicUnit=on
  wires:
  Data Store Read7/1 -> If/1
  If/1 -> If Action Subsystem/Action
  Data Store Read1/1 -> If/2

== system PFC_69C_03_06_V01_3Phase_3_2KW/Calibration,RMS, Fault Protection @5kHz/Voltage sensing ==
  note: Voltage sensing changed to 7, no load Vbulk will trigger Vbulk OVP.
      | Voltage sensing changed to 10, no load Vbulk will not trigger OVP.
  function : TriggerPort  TriggerType=function-call  VariantControl=(inherit)
  Data Store Write16 : DataStoreWrite  DataStoreName=Vmid_ADC  IndexOptions=Index vector (dialog)  Indices=1  OutputSizes=1
  Data Store Write17 : DataStoreWrite  DataStoreName=Vin_ADC_Phase_B  IndexOptions=Index vector (dialog)  Indices=1  OutputSizes=1
  Data Store Write18 : DataStoreWrite  DataStoreName=Vbulk_ADC  IndexOptions=Index vector (dialog)  Indices=1  OutputSizes=1
  Data Store Write5 : DataStoreWrite  DataStoreName=Vin_ADC_Phase_C  IndexOptions=Index vector (dialog)  Indices=1  OutputSizes=1
  Data Store Write7 : DataStoreWrite  DataStoreName=Vin_ADC_Phase_A  IndexOptions=Index vector (dialog)  Indices=1  OutputSizes=1
  Vbulk2 : c2802xlib/ADC  blkParamProc=C2000  ADCModule=1  samplingMode=Single sample mode  ADCResolution=12-bit (Single-ended input)  useSOC1=SOC6  useSOC2=SOC0_SOC1  SOCAcquisitionWindow=10  SOCTriggerSource=Software  SOCInterruptTrigger=No ADCINT  Ts=-1  dType=double  postInterrupt=off  interruptSel=ADCINT1  ADCINTContinuous=off  endma=off  chdma=1  conv1=ADCINA3  conv2=ADCINA0 and ADCINB0  conv1_Type4=ADCIN0  conv2_Type4=ADCIN0 and ADCIN1
      settings: LibrarySourceBlock=c2806xlib/ADC
  Vin5 : c2802xlib/ADC  blkParamProc=C2000  ADCModule=1  samplingMode=Single sample mode  ADCResolution=12-bit (Single-ended input)  useSOC1=SOC3  useSOC2=SOC2_SOC3  SOCAcquisitionWindow=10  SOCTriggerSource=Software  SOCInterruptTrigger=No ADCINT  Ts=-1  dType=double  postInterrupt=off  interruptSel=ADCINT1  ADCINTContinuous=off  endma=off  chdma=1  conv1=ADCINB2  conv2=ADCINA0 and ADCINB0  conv1_Type4=ADCIN0  conv2_Type4=ADCIN0 and ADCIN1
      settings: LibrarySourceBlock=c2806xlib/ADC
  Vin6 : c2802xlib/ADC  blkParamProc=C2000  ADCModule=1  samplingMode=Single sample mode  ADCResolution=12-bit (Single-ended input)  useSOC1=SOC7  useSOC2=SOC6_SOC7  SOCAcquisitionWindow=10  SOCTriggerSource=Software  SOCInterruptTrigger=No ADCINT  Ts=-1  dType=double  postInterrupt=off  interruptSel=ADCINT1  ADCINTContinuous=on  endma=off  chdma=1  conv1=ADCINB0  conv2=ADCINA0 and ADCINB0  conv1_Type4=ADCIN0  conv2_Type4=ADCIN0 and ADCIN1
      settings: LibrarySourceBlock=c2806xlib/ADC
  Vin7 : c2802xlib/ADC  blkParamProc=C2000  ADCModule=1  samplingMode=Single sample mode  ADCResolution=12-bit (Single-ended input)  useSOC1=SOC4  useSOC2=SOC2_SOC3  SOCAcquisitionWindow=10  SOCTriggerSource=Software  SOCInterruptTrigger=No ADCINT  Ts=-1  dType=double  postInterrupt=off  interruptSel=ADCINT1  ADCINTContinuous=off  endma=off  chdma=1  conv1=ADCINB1  conv2=ADCINA0 and ADCINB0  conv1_Type4=ADCIN0  conv2_Type4=ADCIN0 and ADCIN1
      settings: LibrarySourceBlock=c2806xlib/ADC
  Vmid2 : c2802xlib/ADC  blkParamProc=C2000  ADCModule=1  samplingMode=Single sample mode  ADCResolution=12-bit (Single-ended input)  useSOC1=SOC5  useSOC2=SOC0_SOC1  SOCAcquisitionWindow=10  SOCTriggerSource=Software  SOCInterruptTrigger=No ADCINT  Ts=-1  dType=double  postInterrupt=off  interruptSel=ADCINT1  ADCINTContinuous=on  endma=off  chdma=1  conv1=ADCINA4  conv2=ADCINA0 and ADCINB0  conv1_Type4=ADCIN0  conv2_Type4=ADCIN0 and ADCIN1
      settings: LibrarySourceBlock=c2806xlib/ADC
  wires:
  Vin7/1 -> Data Store Write17/1
  Vmid2/1 -> Data Store Write16/1
  Vin6/1 -> Data Store Write5/1
  Vin5/1 -> Data Store Write7/1
  Vbulk2/1 -> Data Store Write18/1

== system PFC_69C_03_06_V01_3Phase_3_2KW/Duty update via UART/Simulink Function ==
  note: Ascii to number
  SCI_Receive : TriggerPort  TriggerType=function-call  IsSimulinkFunction=on  FunctionName=SCI_Receive  FunctionVisibility=scoped  VariantControl=(inherit)
  Constant2 : Constant  Value=48
  Constant3 : Constant  Value=48
  Constant4 : Constant  Value=48
  Demux : Demux  Outputs=3
  Gain2 : Gain  Gain=100
  Gain3 : Gain  Gain=10
  Gain4 : Gain
  SCI Receive : c280xlib/SCI Receive  Priority=2  sciModule=A  dataHead=''  headerCheckMaxCount=16  dataTail=''  dataType=uint8  dataLenOptions=Length via dialog  dataDim=3  maxDataLength=100  initValue=0  errOption=Output custom value  errValue=0  sampleTime=-1  blockingMode=on  timeOut=0.01944  outputStatus=off
      settings: LibrarySourceBlock=c2806xlib/SCI Receive
  Sum2 : Sum  Inputs=|+-
  Sum3 : Sum  Inputs=|+-
  Sum4 : Sum  Inputs=|+-
  Sum5 : Sum  Inputs=|+++  AccumDataTypeStr=double  OutDataTypeStr=double
  y : ArgOut  DisableCoverage=on  ArgumentName=y
  wires:
  Constant4/1 -> Sum4/2
  SCI Receive/1 -> Demux/1
  Gain4/1 -> Sum5/3
  Constant2/1 -> Sum2/2
  Demux/1 -> Sum2/1
  Sum3/1 -> Gain3/1
  Demux/2 -> Sum3/1
  Demux/3 -> Sum4/1
  Sum4/1 -> Gain4/1
  Constant3/1 -> Sum3/2
  Sum2/1 -> Gain2/1
  Gain2/1 -> Sum5/1
  Gain3/1 -> Sum5/2
  Sum5/1 -> y/1

== system PFC_69C_03_06_V01_3Phase_3_2KW/Initialize Function/Subsystem1 ==
  kHz : Inport
  % : Inport  Port=2
  Constant1 : Constant  Value=90E6
  Constant2 : Constant
  Divide : Product  Inputs=*/  RndMeth=Zero  SaturateOnIntegerOverflow=on
  Gain : Gain  Gain=1000
  Gain1 : Gain  Gain=1/100
  Product1 : Product
  Subtract : Sum  Inputs=+-
  Out1 : Outport
  Out2 : Outport  Port=2
  wires:
  kHz/1 -> Gain/1
  Constant1/1 -> Divide/1
  Gain/1 -> Divide/2
  Divide/1 -> Product1/1, Out1/1
  %/1 -> Gain1/1
  Constant2/1 -> Subtract/1
  Gain1/1 -> Subtract/2
  Subtract/1 -> Product1/2
  Product1/1 -> Out2/1

== system PFC_69C_03_06_V01_3Phase_3_2KW/Initialize Function/Subsystem2 ==
  Hz : Inport
  Duty : Inport  Port=2
  128*14 divider : Gain  Gain=1/(128*14)
  Constant1 : Constant  Value=90E6
  Constant2 : Constant
  Divide : Product  Inputs=*/  RndMeth=Zero  SaturateOnIntegerOverflow=on
  Floor : Rounding  Operator=round
  Floor1 : Rounding  Operator=round
  Gain1 : Gain  Gain=1/100
  Product1 : Product
  Subtract : Sum  Inputs=+-
  Out1 : Outport
  Out2 : Outport  Port=2
  wires:
  Duty/1 -> Gain1/1
  Divide/1 -> Floor/1, Product1/1
  Floor1/1 -> Out2/1
  Hz/1 -> 128*14 divider/1
  128*14 divider/1 -> Divide/2
  Constant2/1 -> Subtract/1
  Gain1/1 -> Subtract/2
  Constant1/1 -> Divide/1
  Subtract/1 -> Product1/2
  Product1/1 -> Floor1/1
  Floor/1 -> Out1/1

== system PFC_69C_03_06_V01_3Phase_3_2KW/Initialize Function/Subsystem3 ==
  kHz : Inport
  % : Inport  Port=2
  Constant1 : Constant  Value=90E6
  Constant2 : Constant
  Divide : Product  Inputs=*/  RndMeth=Zero  SaturateOnIntegerOverflow=on
  Gain : Gain  Gain=1000
  Gain1 : Gain  Gain=1/100
  Product1 : Product
  Subtract : Sum  Inputs=+-
  Out1 : Outport
  Out2 : Outport  Port=2
  wires:
  kHz/1 -> Gain/1
  Constant1/1 -> Divide/1
  Gain/1 -> Divide/2
  Divide/1 -> Product1/1, Out1/1
  %/1 -> Gain1/1
  Constant2/1 -> Subtract/1
  Gain1/1 -> Subtract/2
  Subtract/1 -> Product1/2
  Product1/1 -> Out2/1

== system PFC_69C_03_06_V01_3Phase_3_2KW/PWM Update @50KHz/Current loop PWM generation (Control) ==
  function : TriggerPort  TriggerType=function-call  VariantControl=(inherit)
  Data Store Read1 : DataStoreRead  DataStoreName=Relay_started  IndexOptions=Index vector (dialog)  Indices=1  OutputSizes=1
  Data Store Read7 : DataStoreRead  DataStoreName=PFC_en  IndexOptions=Index vector (dialog)  Indices=1  OutputSizes=1
  If : If  NumInputs=2  IfExpression=(u1 ==1) & (u2==1)  ShowElse=off
  If Action Subsystem : Subsystem  TreatAsAtomicUnit=on
  wires:
  Data Store Read7/1 -> If/1
  If/1 -> If Action Subsystem/Action
  Data Store Read1/1 -> If/2
